simulink model "HPWnew"  (R2015a)
settings: Solver=ode45  StartTime=0.0  StopTime=10.0  RelTol=1e-3
undefined symbols (not defined in the file): c1, c2, c3, c4, c5, c6, Hydride, Metal, Nickel, PV1, PV2, PV3
libraries: powerlib x263, electricdrivelib x30, powerlib_meascontrol x15, powerlib_extras x7, re_lib x3, fuzblock x3, simulink x2
(part 1 of 8)
settings Model: Creator=Indhu  LastModifiedBy=Indhu
settings DebuggingCC: SolverPrmCheckMsg=warning

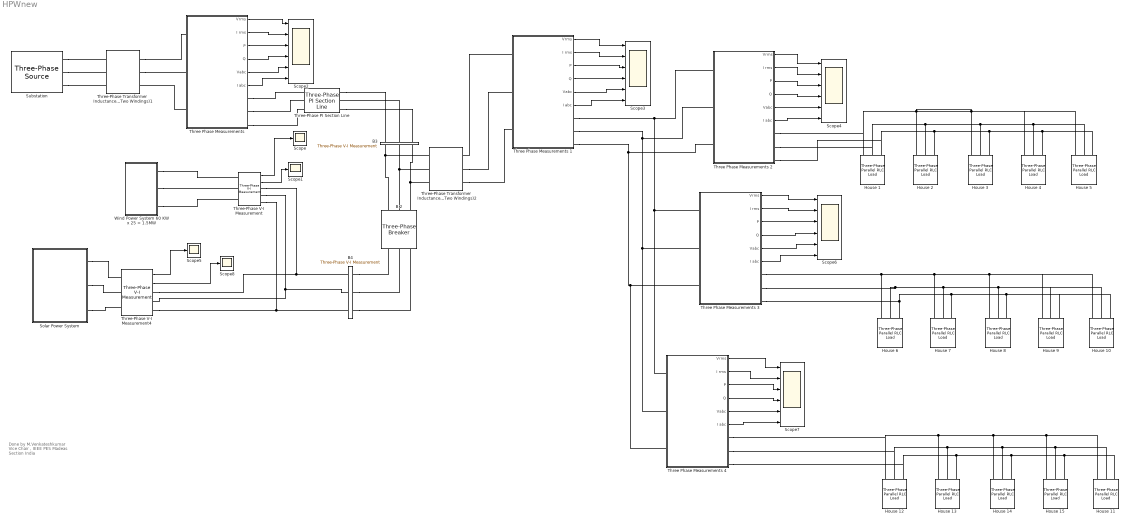
== system HPWnew ==
  note: Done by
      | M.Venkateshkumar
      | Vice Chair , IEEE PES
      | Madeas Section India
  B 2 : powerlib/Elements/Three-Phase Breaker  InitialState=closed  SwitchA=off  SwitchB=off  SwitchC=off  SwitchTimes=[0.001 0.3]  External=off  BreakerResistance=0.001  SnubberResistance=1e6  SnubberCapacitance=inf  Measurements=None
  B3 : powerlib/Measurements/Three-Phase V-I Measurement  VoltageMeasurement=phase-to-ground  SetLabelV=on  LabelV=Vabc_B3  Vpu=off  VpuLL=off  CurrentMeasurement=yes  SetLabelI=on  LabelI=A3  Ipu=off  Pbase=100e6  Vbase=440  OutputType=Magnitude  PhasorSimulation=off  PSBequivalent=0
  B4 : powerlib/Measurements/Three-Phase V-I Measurement  VoltageMeasurement=phase-to-phase  SetLabelV=on  LabelV=Vabc_B4  Vpu=off  VpuLL=off  CurrentMeasurement=yes  SetLabelI=on  LabelI=Iabc_B4  Ipu=off  Pbase=100e6  Vbase=440  OutputType=Magnitude  PhasorSimulation=off  PSBequivalent=0
  House {1..5} (5 alike) : powerlib/Elements/Three-Phase Parallel RLC Load  LConnTagsString=A|B|C  Configuration=Y (grounded)  NominalVoltage=440  NominalFrequency=50  ActivePower=10e2  InductivePower=100  CapacitivePower=0  Measurements=None  LoadType=constant Z
  House {6..10} (5 alike) : powerlib/Elements/Three-Phase Parallel RLC Load  LConnTagsString=A|B|C  Configuration=Y (grounded)  NominalVoltage=440  NominalFrequency=50  ActivePower=10e3  InductivePower=100  CapacitivePower=0  Measurements=None  LoadType=constant Z
  House {11..15} (5 alike) : powerlib/Elements/Three-Phase Parallel RLC Load  LConnTagsString=A|B|C  Configuration=Y (grounded)  NominalVoltage=440  NominalFrequency=50  ActivePower=50e3  InductivePower=100  CapacitivePower=0  Measurements=None  LoadType=constant Z
  Scope{,1,5,8} (4 alike) : Scope
      Scope settings: YMin=-750  YMax=750
      Scope1 settings: YMin=-250  YMax=250  SaveName=ScopeData2
      Scope5 settings: YMin=-600  YMax=550  SaveName=ScopeData8
      Scope8 settings: SaveName=ScopeData9
  Scope{2..4,6..7} (5 alike) : Scope  NumInputPorts=6
      Scope2 settings: TimeRange=1.6  YMin=100~50~-100000~-100000~-500~-500  YMax=300~200~100000~100000~500~500  SaveName=ScopeData3
      Scope3 settings: TimeRange=1.6  YMin=100~50~-100000~-100000~-500~-500  YMax=300~200~100000~100000~500~500  SaveName=ScopeData4
      Scope4 settings: TimeRange=1.6  YMin=100~50~-100000~-100000~-500~-500  YMax=300~200~100000~100000~500~500  SaveName=ScopeData6
      Scope6 settings: TimeRange=1.6  YMin=100~50~-100000~-100000~-500~-500  YMax=300~200~100000~100000~500~500  SaveName=ScopeData7
      Scope7 settings: TimeRange=1.6  YMin=100~50~-100000~-100000~-500~-500  YMax=300~200~100000~100000~500~500  SaveName=ScopeData10
  "Solar Power System " : Subsystem
  "Substation " : powerlib/Electrical Sources/Three-Phase Source  Voltage=(25000)*1.00008  PhaseAngle=0.13223  Frequency=50  InternalConnection=Yg  SpecifyImpedance=on  Resistance=0.8929  Inductance=16.58e-3  ShortCircuitLevel=100e6  BaseVoltage=63510.4  XRratio=7  BusType=swing  Pref=0  Qref=0  Qmin=-inf  Qmax=inf
  "Three Phase Measurements " : Subsystem
  Three Phase Measurements 1 : Subsystem
  Three Phase Measurements 2 : Subsystem
  Three Phase Measurements 3 : Subsystem
  Three Phase Measurements 4 : Subsystem
  Three-Phase PI Section Line : powerlib/Elements/Three-Phase PI Section Line  LConnTagsString=a|b|c  RConnTagsString=A|B|C  Frequency=50  Resistances=[ 0.01273 0.3864]  Inductances="[ 0.9337e-3  4.1264e-3]"  Capacitances=[12.74e-9 7.751e-9]  Length=10
  Three-Phase V-I Measurement : powerlib/Measurements/Three-Phase V-I Measurement  VoltageMeasurement=phase-to-ground  SetLabelV=off  LabelV=Vabc  Vpu=off  VpuLL=off  CurrentMeasurement=yes  SetLabelI=off  LabelI=Iabc  Ipu=off  Pbase=100e6  Vbase=500e3  OutputType=Complex  PhasorSimulation=off  PSBequivalent=0
  Three-Phase V-I Measurement4 : powerlib/Measurements/Three-Phase V-I Measurement  VoltageMeasurement=phase-to-ground  SetLabelV=off  LabelV=Vabc  Vpu=off  VpuLL=off  CurrentMeasurement=yes  SetLabelI=off  LabelI=Iabc  Ipu=off  Pbase=100e6  Vbase=500e3  OutputType=Complex  PhasorSimulation=off  PSBequivalent=0
  Three-Phase Transformer Inductance Matrix Type (Two Windings)1 : powerlib/Elements/Three-Phase Transformer Inductance Matrix Type (Two Windings)  CoreType=Three-limb or five-limb core  Winding1Connection=Yg  Winding2Connection=Yg  AutoTransformer=off  Measurements=None  NominalPower=[100e3 50]  VLLnom=[63510.4 600]  WindingResistances=[0.01 0.01]  NoLoadIexcPos=2  NoLoadPlossPos=1000  ShortCircuitReactancePos=0.06  ShortCircuitReactancePosAuto=0.06  NoLoadIexcZero=100  NoLoadPlossZero=1500  ShortCircuitReactanceZero=0.03  ShortCircuitReactanceZeroAuto=0.03
  Three-Phase Transformer Inductance Matrix Type (Two Windings)2 : powerlib/Elements/Three-Phase Transformer Inductance Matrix Type (Two Windings)  CoreType=Three-limb or five-limb core  Winding1Connection=Yg  Winding2Connection=Yg  AutoTransformer=off  Measurements=None  NominalPower=[100e3 50]  VLLnom=[63510.4 600]  WindingResistances=[0.01 0.01]  NoLoadIexcPos=2  NoLoadPlossPos=1000  ShortCircuitReactancePos=0.06  ShortCircuitReactancePosAuto=0.06  NoLoadIexcZero=100  NoLoadPlossZero=1500  ShortCircuitReactanceZero=0.03  ShortCircuitReactanceZeroAuto=0.03
  Wind Power System 60 KW x 25 = 1.5MW : Subsystem
  wires:
  Three-Phase V-I Measurement/1 -> Scope/1
  Three-Phase V-I Measurement/2 -> Scope1/1
  Three-Phase V-I Measurement4/1 -> Scope5/1
  Three-Phase V-I Measurement4/2 -> Scope8/1
  "Three Phase Measurements "/3(P) -> Scope2/3
  "Three Phase Measurements "/4(Q) -> Scope2/4
  "Three Phase Measurements "/2(I rms) -> Scope2/2
  "Three Phase Measurements "/5(Vabc) -> Scope2/5
  "Three Phase Measurements "/1(Vrms) -> Scope2/1
  "Three Phase Measurements "/6(I abc) -> Scope2/6
  Three Phase Measurements 1/3(P) -> Scope3/3
  Three Phase Measurements 1/4(Q) -> Scope3/4
  Three Phase Measurements 1/2(I rms) -> Scope3/2
  Three Phase Measurements 1/5(Vabc) -> Scope3/5
  Three Phase Measurements 1/1(Vrms) -> Scope3/1
  Three Phase Measurements 1/6(I abc) -> Scope3/6
  Three Phase Measurements 2/3(P) -> Scope4/3
  Three Phase Measurements 2/4(Q) -> Scope4/4
  Three Phase Measurements 2/2(I rms) -> Scope4/2
  Three Phase Measurements 2/5(Vabc) -> Scope4/5
  Three Phase Measurements 2/1(Vrms) -> Scope4/1
  Three Phase Measurements 2/6(I abc) -> Scope4/6
  Three Phase Measurements 3/3(P) -> Scope6/3
  Three Phase Measurements 3/4(Q) -> Scope6/4
  Three Phase Measurements 3/2(I rms) -> Scope6/2
  Three Phase Measurements 3/5(Vabc) -> Scope6/5
  Three Phase Measurements 3/1(Vrms) -> Scope6/1
  Three Phase Measurements 3/6(I abc) -> Scope6/6
  Three Phase Measurements 4/3(P) -> Scope7/3
  Three Phase Measurements 4/4(Q) -> Scope7/4
  Three Phase Measurements 4/2(I rms) -> Scope7/2
  Three Phase Measurements 4/5(Vabc) -> Scope7/5
  Three Phase Measurements 4/1(Vrms) -> Scope7/1
  Three Phase Measurements 4/6(I abc) -> Scope7/6
  connections:
  B 2/LConn1 -- Three-Phase Transformer Inductance Matrix Type (Two Windings)2/LConn1 -- B3/LConn1
  B 2/LConn2 -- Three-Phase Transformer Inductance Matrix Type (Two Windings)2/LConn2 -- B3/LConn2
  B 2/LConn3 -- Three-Phase Transformer Inductance Matrix Type (Two Windings)2/LConn3 -- B3/LConn3
  B4/LConn3 -- B 2/RConn3
  B4/LConn1 -- B 2/RConn1
  B4/LConn2 -- B 2/RConn2
  "Solar Power System "/RConn2 -- Three-Phase V-I Measurement4/LConn2
  "Solar Power System "/RConn3 -- Three-Phase V-I Measurement4/LConn3
  "Solar Power System "/RConn1 -- Three-Phase V-I Measurement4/LConn1
  "Three Phase Measurements "/LConn3 -- Three-Phase Transformer Inductance Matrix Type (Two Windings)1/RConn3
  Three-Phase Transformer Inductance Matrix Type (Two Windings)1/RConn2 -- "Three Phase Measurements "/LConn2
  Three-Phase Transformer Inductance Matrix Type (Two Windings)1/RConn1 -- "Three Phase Measurements "/LConn1
  "Substation "/RConn1 -- Three-Phase Transformer Inductance Matrix Type (Two Windings)1/LConn1
  "Substation "/RConn2 -- Three-Phase Transformer Inductance Matrix Type (Two Windings)1/LConn2
  "Substation "/RConn3 -- Three-Phase Transformer Inductance Matrix Type (Two Windings)1/LConn3
  Three-Phase PI Section Line/RConn1 -- B3/RConn1
  B3/RConn2 -- Three-Phase PI Section Line/RConn2
  Three-Phase PI Section Line/RConn3 -- B3/RConn3
  Three-Phase V-I Measurement/RConn1 -- Three-Phase V-I Measurement4/RConn1 -- B4/RConn1
  Three-Phase V-I Measurement/RConn2 -- Three-Phase V-I Measurement4/RConn2 -- B4/RConn2
  Three-Phase V-I Measurement/RConn3 -- Three-Phase V-I Measurement4/RConn3 -- B4/RConn3
  House 4/LConn1 -- House 5/LConn1 -- House 3/LConn1 -- House 1/LConn1 -- Three Phase Measurements 2/RConn1 -- House 2/LConn1
  House 11/LConn2 -- House 15/LConn2 -- House 14/LConn2 -- Three Phase Measurements 4/RConn2 -- House 12/LConn2 -- House 13/LConn2
  House 11/LConn3 -- House 15/LConn3 -- House 14/LConn3 -- Three Phase Measurements 4/RConn3 -- House 12/LConn3 -- House 13/LConn3
  "Three Phase Measurements "/RConn1 -- Three-Phase PI Section Line/LConn1
  "Three Phase Measurements "/RConn2 -- Three-Phase PI Section Line/LConn2
  "Three Phase Measurements "/RConn3 -- Three-Phase PI Section Line/LConn3
  Three-Phase Transformer Inductance Matrix Type (Two Windings)2/RConn1 -- Three Phase Measurements 1/LConn1
  Three-Phase Transformer Inductance Matrix Type (Two Windings)2/RConn2 -- Three Phase Measurements 1/LConn2
  Three-Phase Transformer Inductance Matrix Type (Two Windings)2/RConn3 -- Three Phase Measurements 1/LConn3
  Wind Power System 60 KW x 25 = 1.5MW/RConn2 -- Three-Phase V-I Measurement/LConn2
  Wind Power System 60 KW x 25 = 1.5MW/RConn1 -- Three-Phase V-I Measurement/LConn1
  Wind Power System 60 KW x 25 = 1.5MW/RConn3 -- Three-Phase V-I Measurement/LConn3
  House 4/LConn3 -- House 1/LConn3 -- Three Phase Measurements 2/RConn3 -- House 2/LConn3 -- House 3/LConn3 -- House 5/LConn3
  House 4/LConn2 -- House 1/LConn2 -- Three Phase Measurements 2/RConn2 -- House 2/LConn2 -- House 3/LConn2 -- House 5/LConn2
  House 8/LConn1 -- House 10/LConn1 -- House 9/LConn1 -- House 7/LConn1 -- House 6/LConn1 -- Three Phase Measurements 3/RConn1
  House 7/LConn2 -- House 8/LConn2 -- House 10/LConn2 -- House 9/LConn2 -- Three Phase Measurements 3/RConn2 -- House 6/LConn2
  House 15/LConn1 -- House 11/LConn1 -- House 14/LConn1 -- Three Phase Measurements 4/RConn1 -- House 12/LConn1 -- House 13/LConn1
  House 7/LConn3 -- House 8/LConn3 -- House 10/LConn3 -- House 9/LConn3 -- House 6/LConn3 -- Three Phase Measurements 3/RConn3
  Three Phase Measurements 3/LConn1 -- Three Phase Measurements 2/LConn1 -- Three Phase Measurements 1/RConn1 -- Three Phase Measurements 4/LConn1
  Three Phase Measurements 3/LConn2 -- Three Phase Measurements 2/LConn2 -- Three Phase Measurements 1/RConn2 -- Three Phase Measurements 4/LConn2
  Three Phase Measurements 3/LConn3 -- Three Phase Measurements 4/LConn3 -- Three Phase Measurements 2/LConn3 -- Three Phase Measurements 1/RConn3

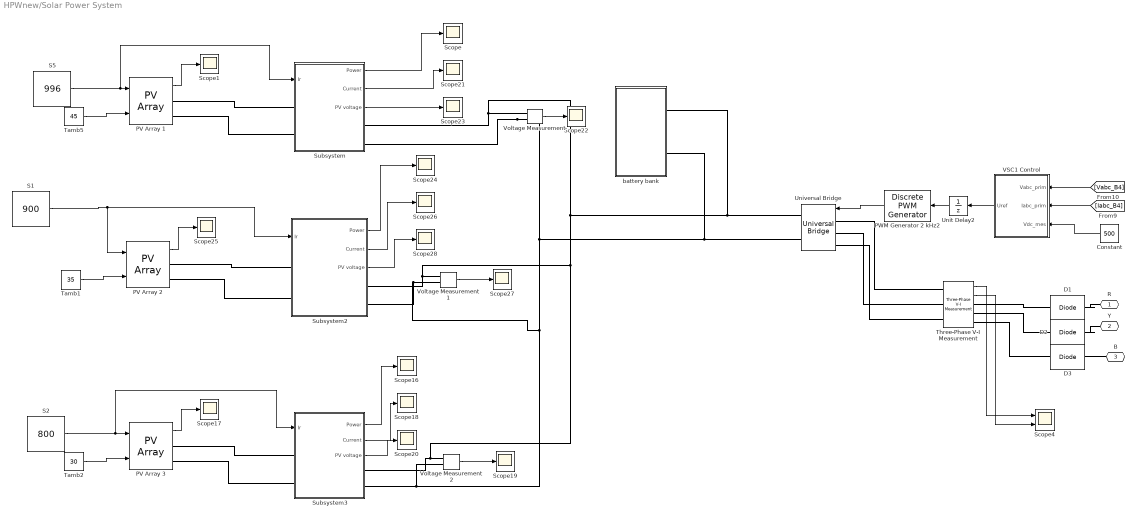
== system HPWnew/Solar Power System  ==
  Constant : Constant  Value=500
  D1 : powerlib/Power Electronics/Diode  Ron=0.001  Lon=0  Vf=0.1  IC=0  UseSnubber=off  Rs=50000  Cs=250e-12  Measurements=off
  D2 : powerlib/Power Electronics/Diode  Ron=0.001  Lon=0  Vf=0.1  IC=0  UseSnubber=off  Rs=50000  Cs=250e-12  Measurements=off
  D3 : powerlib/Power Electronics/Diode  Ron=0.001  Lon=0  Vf=0.1  IC=0  UseSnubber=off  Rs=50000  Cs=250e-12  Measurements=off
  PV Array 1 : re_lib/Solar/PV Array  Npar=3  Nser=1  PlotType=array @ 25 deg.C & specified irradiances  S_vec="[ 1000  500  100 ]"  Temp_C_vec="[ 45 25  ]"  ModuleName=User-defined  PlotWhenSelected=on  Pm=276.21  Ncell=36  Voc=41.8  Isc=7.4  Vm=40.5  Im=6.82  beta_Voc_pc=-0.365  alpha_Isc_pc=0.0445  beta_Voc=-0.15257  alpha_Isc=0.003293  IL=7.4001  I0=1.6325e-15  nI=1.3667  Rsh=139.6555  Rs=0.080363  BAL=off  Tc=1e-6  Tfilter=10
  PV Array 2 : re_lib/Solar/PV Array  Npar=3  Nser=1  PlotType=array @ 25 deg.C & specified irradiances  S_vec="[ 1000  500  100 ]"  Temp_C_vec="[ 45 25  ]"  ModuleName=User-defined  PlotWhenSelected=on  Pm=276.21  Ncell=36  Voc=41.8  Isc=7.4  Vm=40.5  Im=6.82  beta_Voc_pc=-0.365  alpha_Isc_pc=0.0445  beta_Voc=-0.15257  alpha_Isc=0.003293  IL=7.4001  I0=1.6325e-15  nI=1.3667  Rsh=139.6555  Rs=0.080363  BAL=off  Tc=1e-6  Tfilter=10
  PV Array 3 : re_lib/Solar/PV Array  Npar=3  Nser=1  PlotType=array @ 25 deg.C & specified irradiances  S_vec="[ 1000  500  100 ]"  Temp_C_vec="[ 45 25  ]"  ModuleName=User-defined  PlotWhenSelected=on  Pm=276.21  Ncell=36  Voc=41.8  Isc=7.4  Vm=40.5  Im=6.82  beta_Voc_pc=-0.365  alpha_Isc_pc=0.0445  beta_Voc=-0.15257  alpha_Isc=0.003293  IL=7.4001  I0=1.6325e-15  nI=1.3667  Rsh=139.6555  Rs=0.080363  BAL=off  Tc=1e-6  Tfilter=10
  PWM Generator 2 kHz2 : powerlib_extras/Discrete  Control Blocks/Discrete PWM Generator  GeneratorMode="3-arm  bridge (6 pulses)"  Fc=33*50  Ts=1  Internal=off  mIndex=0.4  Freq=60  Phase=0
  S1 : Constant  Value=900
  S2 : Constant  Value=800
  S5 : Constant  Value=996
  Scope{,1,16..28} (15 alike) : Scope
      Scope settings: YMin=1000  YMax=2200  SaveName=ScopeData5
      Scope1 settings: YMin=3.1175  YMax=3.145  SaveName=ScopeData24  MaxDataPoints=50000000
      Scope16 settings: YMin=-125  YMax=175  SaveName=ScopeData19
      Scope17 settings: YMin=3.1175  YMax=3.145  SaveName=ScopeData20  MaxDataPoints=50000000
      Scope18 settings: YMin=1.845  YMax=1.857  SaveName=ScopeData21
      Scope19 settings: YMin=190.2  YMax=191.4  SaveName=ScopeData22
      Scope20 settings: YMin=34.5  YMax=41  SaveName=ScopeData23
      Scope21 settings: YMin=1.845  YMax=1.857  SaveName=ScopeData25
      Scope22 settings: YMin=499.8  YMax=500.2  SaveName=ScopeData26
      Scope23 settings: YMin=0  YMax=225  SaveName=ScopeData27
      Scope24 settings: YMin=-1000  YMax=10000  SaveName=ScopeData28
      Scope25 settings: YMin=3.1175  YMax=3.145  SaveName=ScopeData29  MaxDataPoints=50000000
      Scope26 settings: YMin=1.845  YMax=1.857  SaveName=ScopeData30
      Scope27 settings: YMin=499.8  YMax=500.2  SaveName=ScopeData31
      Scope28 settings: YMin=0  YMax=200  SaveName=ScopeData18
  Scope4 : Scope  NumInputPorts=2
      settings: ShowLegends=on  YMin=-950~-0.025  YMax=-100~0.5  SaveName=MLFCDSTAT
  Subsystem : Subsystem
  Subsystem2 : Subsystem
  Subsystem3 : Subsystem
  Tamb1 : Constant  Value=35
  Tamb2 : Constant  Value=30
  Tamb5 : Constant  Value=45
  Three-Phase V-I Measurement : powerlib/Measurements/Three-Phase V-I Measurement  VoltageMeasurement=phase-to-ground  SetLabelV=off  LabelV=Vabc  Vpu=off  VpuLL=off  CurrentMeasurement=yes  SetLabelI=off  LabelI=Iabc  Ipu=off  Pbase=100e6  Vbase=500e3  OutputType=Complex  PhasorSimulation=off  PSBequivalent=0
  Unit Delay2 : UnitDelay
  Universal Bridge : powerlib/Power Electronics/Universal Bridge  Arms=3  SnubberResistance=1e5  SnubberCapacitance=inf  Device=MOSFET / Diodes  Ron=1e-3  Lon=0  ForwardVoltages="[  0  0  ]"  ForwardVoltage=0  GTOparameters=[ 10e-6 , 20e-6 ]  IGBTparameters=[ 1e-6 , 2e-6 ]  Measurements=None  Measurements_2=None  converterType=Rectifier
  VSC1 Control : Subsystem  mask(VSC Main Controller){nom=[ 50e3  50 ], Vnom=[ 6350.9 254.03 ], Vnom_dc=500, RLxfo=[0.008  0.04 ], RLchoke=[2e-3*(2*pi*60)/50   2e-3], K_VDCreg=[7  800], K_Ireg=[0.3 20]*1.5, Ts=1}
      mask prompts: nom "Nominal power and frequency [ Pnom(VA)  Fnom(Hz) ]:"; Vnom "Nominal primary and secondary voltages (Vrms LL) [ Vnom_prim   Vnom_sec ]:"; Vnom_dc "Nominal DC bus voltage (V):"; RLxfo "Total transformer leakage impedance (pu/Pnom) [ Rxfo  Lxf ]"; RLchoke "Choke impedance [ R(ohm) L(H) ]"; K_VDCreg "VDC regultator gains [ Kp  Ki ]:"; K_Ireg "Current regulator gains [ Kp  Ki ]:"; Ts "Sample time"
      mask init:
      | Pnom=nom(1);
      | Fnom=nom(2);
      | Vnom_prim=Vnom(1);
      | Vnom_sec=Vnom(2);
      | Zbase=Vnom_sec^2/Pnom;
      | Rtot_pu=RLxfo(1) + RLchoke(1)/Zbase;
      | Ltot_pu=RLxfo(2) + RLchoke(2)/(Zbase/(2*pi*Fnom));
      | Kp_VDCreg=K_VDCreg(1);
      | Ki_VDCreg=K_VDCreg(2);
      | Kp_Ireg=K_Ireg(1);
      | Ki_Ireg=K_Ireg(2);
      | Vdc_ref=Vnom_dc;
      | % Used to determine initial value of Boost Control (MPPT)
      | assignin('base','Vdc_ref_Inv',Vdc_ref);
  Voltage Measurement : powerlib/Measurements/Voltage Measurement  PhasorSimulation=off  OutputType=Complex  PSBequivalent=0
  Voltage Measurement1 : powerlib/Measurements/Voltage Measurement  PhasorSimulation=off  OutputType=Complex  PSBequivalent=0
  Voltage Measurement2 : powerlib/Measurements/Voltage Measurement  PhasorSimulation=off  OutputType=Complex  PSBequivalent=0
  "battery bank " : Subsystem
  R : PMIOPort  Port=1  Side=Right
  Y : PMIOPort  Port=2  Side=Right
  B : PMIOPort  Port=3  Side=Right
  wires:
  [Vabc_B4] -> VSC1 Control/1(Vabc_prim)
  [Iabc_B4] -> VSC1 Control/2(Iabc_prim)
  PWM Generator 2 kHz2/1 -> Universal Bridge/1
  Constant/1 -> VSC1 Control/3(Vdc_mes)
  Three-Phase V-I Measurement/1 -> Scope4/1
  Three-Phase V-I Measurement/2 -> Scope4/2
  Unit Delay2/1 -> PWM Generator 2 kHz2/1
  VSC1 Control/1(Uref) -> Unit Delay2/1
  Tamb5/1 -> PV Array 1/2
  PV Array 1/1 -> Scope1/1
  Subsystem/1(Power) -> Scope/1
  Subsystem/2("Current ") -> Scope21/1
  Voltage Measurement/1 -> Scope22/1
  Subsystem/3("PV voltage ") -> Scope23/1
  S1/1 -> Subsystem2/1(Ir), PV Array 2/1
  Tamb1/1 -> PV Array 2/2
  PV Array 2/1 -> Scope25/1
  Subsystem2/1(Power) -> Scope24/1
  Subsystem2/2("Current ") -> Scope26/1
  Voltage Measurement1/1 -> Scope27/1
  Subsystem2/3("PV voltage ") -> Scope28/1
  Tamb2/1 -> PV Array 3/2
  PV Array 3/1 -> Scope17/1
  Subsystem3/1(Power) -> Scope16/1
  Subsystem3/2("Current ") -> Scope18/1
  Voltage Measurement2/1 -> Scope19/1
  Subsystem3/3("PV voltage ") -> Scope20/1
  S5/1 -> Subsystem/1(Ir), PV Array 1/1
  S2/1 -> Subsystem3/1(Ir), PV Array 3/1
  connections:
  Three-Phase V-I Measurement/LConn1 -- Universal Bridge/LConn1
  Three-Phase V-I Measurement/LConn2 -- Universal Bridge/LConn2
  Three-Phase V-I Measurement/RConn2 -- D2/LConn1
  D3/RConn1 -- B/RConn1
  D2/RConn1 -- Y/RConn1
  Three-Phase V-I Measurement/LConn3 -- Universal Bridge/LConn3
  Three-Phase V-I Measurement/RConn1 -- D1/LConn1
  D1/RConn1 -- R/RConn1
  Three-Phase V-I Measurement/RConn3 -- D3/LConn1
  Voltage Measurement2/LConn1 -- Subsystem3/RConn1 -- "battery bank "/RConn1 -- Universal Bridge/RConn1 -- Subsystem/RConn1 -- Voltage Measurement/LConn1 -- Subsystem2/RConn1 -- Voltage Measurement1/LConn1
  Subsystem3/RConn2 -- Voltage Measurement2/LConn2 -- "battery bank "/RConn2 -- Universal Bridge/RConn2 -- Subsystem/RConn2 -- Voltage Measurement/LConn2 -- Subsystem2/RConn2 -- Voltage Measurement1/LConn2
  PV Array 2/RConn2 -- Subsystem2/LConn2
  PV Array 2/RConn1 -- Subsystem2/LConn1
  PV Array 1/RConn2 -- Subsystem/LConn2
  PV Array 1/RConn1 -- Subsystem/LConn1
  PV Array 3/RConn2 -- Subsystem3/LConn2
  PV Array 3/RConn1 -- Subsystem3/LConn1

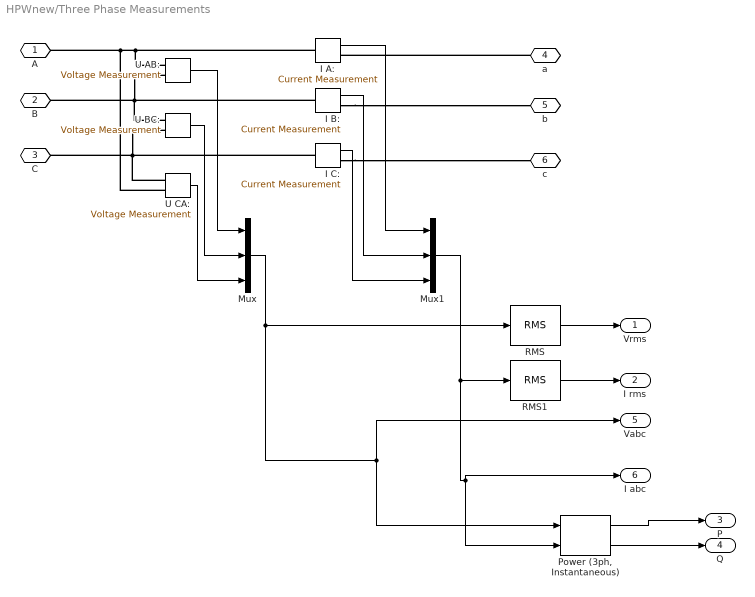
== system HPWnew/Three Phase Measurements  ==
  I A: : powerlib/Measurements/Current Measurement  PhasorSimulation=off  OutputType=Complex  PSBequivalent=0
  I B: : powerlib/Measurements/Current Measurement  PhasorSimulation=off  OutputType=Complex  PSBequivalent=0
  I C: : powerlib/Measurements/Current Measurement  PhasorSimulation=off  OutputType=Complex  PSBequivalent=0
  Mux : Mux  Inputs=3
  Mux1 : Mux  Inputs=3
  "Power (3ph, Instantaneous)" : powerlib_meascontrol/Measurements/Power (3ph, Instantaneous)
  RMS : powerlib_meascontrol/Measurements/RMS  TrueRMS=on  Freq=60  RMSInit=120  Ts=0
  RMS1 : powerlib_meascontrol/Measurements/RMS  TrueRMS=on  Freq=60  RMSInit=120  Ts=0
  U AB: : powerlib/Measurements/Voltage Measurement  PhasorSimulation=off  OutputType=Complex  PSBequivalent=0
  U BC: : powerlib/Measurements/Voltage Measurement  PhasorSimulation=off  OutputType=Complex  PSBequivalent=0
  U CA: : powerlib/Measurements/Voltage Measurement  PhasorSimulation=off  OutputType=Complex  PSBequivalent=0
  A : PMIOPort  Port=1  Side=Left
  B : PMIOPort  Port=2  Side=Left
  C : PMIOPort  Port=3  Side=Left
  a : PMIOPort  Port=4  Side=Right
  b : PMIOPort  Port=5  Side=Right
  c : PMIOPort  Port=6  Side=Right
  Vrms : Outport
  I rms : Outport  Port=2
  P : Outport  Port=3
  Q : Outport  Port=4
  Vabc : Outport  Port=5
  I abc : Outport  Port=6
  wires:
  I A:/1 -> Mux1/1
  Mux/1 -> Vabc/1, "Power (3ph, Instantaneous)"/1, RMS/1
  I C:/1 -> Mux1/3
  I B:/1 -> Mux1/2
  "Power (3ph, Instantaneous)"/2 -> Q/1
  Mux1/1 -> "Power (3ph, Instantaneous)"/2, I abc/1, RMS1/1
  U CA:/1 -> Mux/3
  U AB:/1 -> Mux/1
  U BC:/1 -> Mux/2
  RMS1/1 -> I rms/1
  RMS/1 -> Vrms/1
  "Power (3ph, Instantaneous)"/1 -> P/1
  connections:
  I C:/RConn1 -- c/RConn1
  a/RConn1 -- I A:/RConn1
  U CA:/LConn2 -- I A:/LConn1 -- U AB:/LConn1 -- A/RConn1
  I C:/LConn1 -- U BC:/LConn2 -- U CA:/LConn1 -- C/RConn1
  I B:/LConn1 -- U AB:/LConn2 -- U BC:/LConn1 -- B/RConn1
  I B:/RConn1 -- b/RConn1

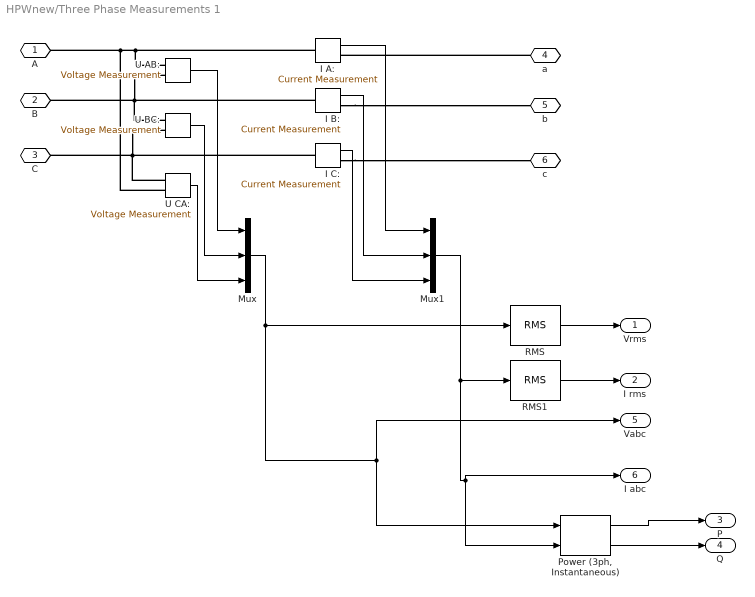
== system HPWnew/Three Phase Measurements 1 ==
  I A: : powerlib/Measurements/Current Measurement  PhasorSimulation=off  OutputType=Complex  PSBequivalent=0
  I B: : powerlib/Measurements/Current Measurement  PhasorSimulation=off  OutputType=Complex  PSBequivalent=0
  I C: : powerlib/Measurements/Current Measurement  PhasorSimulation=off  OutputType=Complex  PSBequivalent=0
  Mux : Mux  Inputs=3
  Mux1 : Mux  Inputs=3
  "Power (3ph, Instantaneous)" : powerlib_meascontrol/Measurements/Power (3ph, Instantaneous)
  RMS : powerlib_meascontrol/Measurements/RMS  TrueRMS=on  Freq=60  RMSInit=120  Ts=0
  RMS1 : powerlib_meascontrol/Measurements/RMS  TrueRMS=on  Freq=60  RMSInit=120  Ts=0
  U AB: : powerlib/Measurements/Voltage Measurement  PhasorSimulation=off  OutputType=Complex  PSBequivalent=0
  U BC: : powerlib/Measurements/Voltage Measurement  PhasorSimulation=off  OutputType=Complex  PSBequivalent=0
  U CA: : powerlib/Measurements/Voltage Measurement  PhasorSimulation=off  OutputType=Complex  PSBequivalent=0
  A : PMIOPort  Port=1  Side=Left
  B : PMIOPort  Port=2  Side=Left
  C : PMIOPort  Port=3  Side=Left
  a : PMIOPort  Port=4  Side=Right
  b : PMIOPort  Port=5  Side=Right
  c : PMIOPort  Port=6  Side=Right
  Vrms : Outport
  I rms : Outport  Port=2
  P : Outport  Port=3
  Q : Outport  Port=4
  Vabc : Outport  Port=5
  I abc : Outport  Port=6
  wires:
  "Power (3ph, Instantaneous)"/1 -> P/1
  RMS/1 -> Vrms/1
  RMS1/1 -> I rms/1
  U BC:/1 -> Mux/2
  U AB:/1 -> Mux/1
  U CA:/1 -> Mux/3
  Mux1/1 -> RMS1/1, I abc/1, "Power (3ph, Instantaneous)"/2
  "Power (3ph, Instantaneous)"/2 -> Q/1
  I B:/1 -> Mux1/2
  I C:/1 -> Mux1/3
  Mux/1 -> RMS/1, "Power (3ph, Instantaneous)"/1, Vabc/1
  I A:/1 -> Mux1/1
  connections:
  I B:/RConn1 -- b/RConn1
  B/RConn1 -- U BC:/LConn1 -- U AB:/LConn2 -- I B:/LConn1
  C/RConn1 -- U CA:/LConn1 -- U BC:/LConn2 -- I C:/LConn1
  A/RConn1 -- U AB:/LConn1 -- I A:/LConn1 -- U CA:/LConn2
  a/RConn1 -- I A:/RConn1
  I C:/RConn1 -- c/RConn1

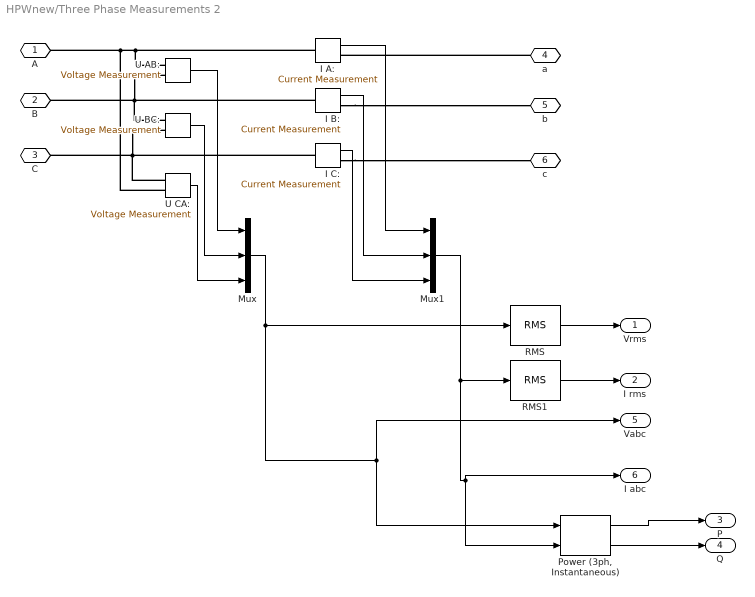
== system HPWnew/Three Phase Measurements 2 ==
  I A: : powerlib/Measurements/Current Measurement  PhasorSimulation=off  OutputType=Complex  PSBequivalent=0
  I B: : powerlib/Measurements/Current Measurement  PhasorSimulation=off  OutputType=Complex  PSBequivalent=0
  I C: : powerlib/Measurements/Current Measurement  PhasorSimulation=off  OutputType=Complex  PSBequivalent=0
  Mux : Mux  Inputs=3
  Mux1 : Mux  Inputs=3
  "Power (3ph, Instantaneous)" : powerlib_meascontrol/Measurements/Power (3ph, Instantaneous)
  RMS : powerlib_meascontrol/Measurements/RMS  TrueRMS=on  Freq=60  RMSInit=120  Ts=0
  RMS1 : powerlib_meascontrol/Measurements/RMS  TrueRMS=on  Freq=60  RMSInit=120  Ts=0
  U AB: : powerlib/Measurements/Voltage Measurement  PhasorSimulation=off  OutputType=Complex  PSBequivalent=0
  U BC: : powerlib/Measurements/Voltage Measurement  PhasorSimulation=off  OutputType=Complex  PSBequivalent=0
  U CA: : powerlib/Measurements/Voltage Measurement  PhasorSimulation=off  OutputType=Complex  PSBequivalent=0
  A : PMIOPort  Port=1  Side=Left
  B : PMIOPort  Port=2  Side=Left
  C : PMIOPort  Port=3  Side=Left
  a : PMIOPort  Port=4  Side=Right
  b : PMIOPort  Port=5  Side=Right
  c : PMIOPort  Port=6  Side=Right
  Vrms : Outport
  I rms : Outport  Port=2
  P : Outport  Port=3
  Q : Outport  Port=4
  Vabc : Outport  Port=5
  I abc : Outport  Port=6
  wires:
  I A:/1 -> Mux1/1
  Mux/1 -> Vabc/1, "Power (3ph, Instantaneous)"/1, RMS/1
  I C:/1 -> Mux1/3
  I B:/1 -> Mux1/2
  "Power (3ph, Instantaneous)"/2 -> Q/1
  Mux1/1 -> "Power (3ph, Instantaneous)"/2, I abc/1, RMS1/1
  U CA:/1 -> Mux/3
  U AB:/1 -> Mux/1
  U BC:/1 -> Mux/2
  RMS1/1 -> I rms/1
  RMS/1 -> Vrms/1
  "Power (3ph, Instantaneous)"/1 -> P/1
  connections:
  I C:/RConn1 -- c/RConn1
  a/RConn1 -- I A:/RConn1
  U CA:/LConn2 -- I A:/LConn1 -- U AB:/LConn1 -- A/RConn1
  I C:/LConn1 -- U BC:/LConn2 -- U CA:/LConn1 -- C/RConn1
  I B:/LConn1 -- U AB:/LConn2 -- U BC:/LConn1 -- B/RConn1
  I B:/RConn1 -- b/RConn1

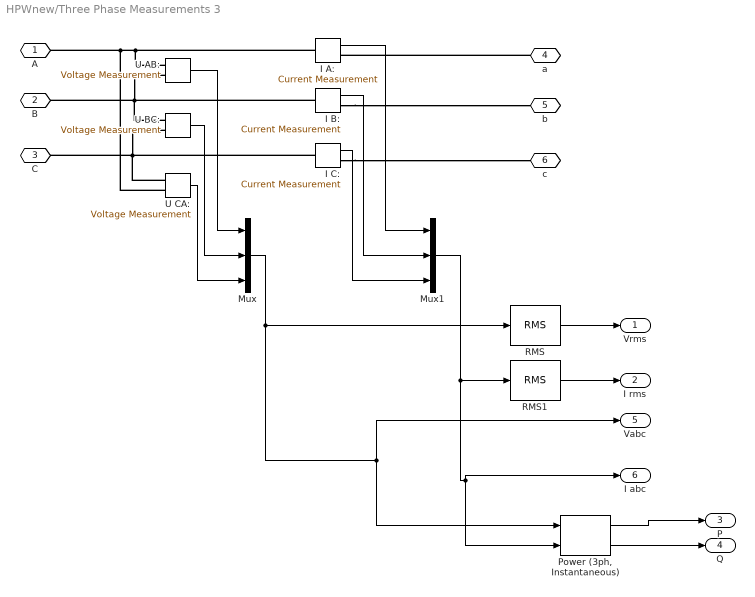
== system HPWnew/Three Phase Measurements 3 ==
  I A: : powerlib/Measurements/Current Measurement  PhasorSimulation=off  OutputType=Complex  PSBequivalent=0
  I B: : powerlib/Measurements/Current Measurement  PhasorSimulation=off  OutputType=Complex  PSBequivalent=0
  I C: : powerlib/Measurements/Current Measurement  PhasorSimulation=off  OutputType=Complex  PSBequivalent=0
  Mux : Mux  Inputs=3
  Mux1 : Mux  Inputs=3
  "Power (3ph, Instantaneous)" : powerlib_meascontrol/Measurements/Power (3ph, Instantaneous)
  RMS : powerlib_meascontrol/Measurements/RMS  TrueRMS=on  Freq=60  RMSInit=120  Ts=0
  RMS1 : powerlib_meascontrol/Measurements/RMS  TrueRMS=on  Freq=60  RMSInit=120  Ts=0
  U AB: : powerlib/Measurements/Voltage Measurement  PhasorSimulation=off  OutputType=Complex  PSBequivalent=0
  U BC: : powerlib/Measurements/Voltage Measurement  PhasorSimulation=off  OutputType=Complex  PSBequivalent=0
  U CA: : powerlib/Measurements/Voltage Measurement  PhasorSimulation=off  OutputType=Complex  PSBequivalent=0
  A : PMIOPort  Port=1  Side=Left
  B : PMIOPort  Port=2  Side=Left
  C : PMIOPort  Port=3  Side=Left
  a : PMIOPort  Port=4  Side=Right
  b : PMIOPort  Port=5  Side=Right
  c : PMIOPort  Port=6  Side=Right
  Vrms : Outport
  I rms : Outport  Port=2
  P : Outport  Port=3
  Q : Outport  Port=4
  Vabc : Outport  Port=5
  I abc : Outport  Port=6
  wires:
  "Power (3ph, Instantaneous)"/1 -> P/1
  RMS/1 -> Vrms/1
  RMS1/1 -> I rms/1
  U BC:/1 -> Mux/2
  U AB:/1 -> Mux/1
  U CA:/1 -> Mux/3
  Mux1/1 -> RMS1/1, I abc/1, "Power (3ph, Instantaneous)"/2
  "Power (3ph, Instantaneous)"/2 -> Q/1
  I B:/1 -> Mux1/2
  I C:/1 -> Mux1/3
  Mux/1 -> RMS/1, "Power (3ph, Instantaneous)"/1, Vabc/1
  I A:/1 -> Mux1/1
  connections:
  I B:/RConn1 -- b/RConn1
  B/RConn1 -- U BC:/LConn1 -- U AB:/LConn2 -- I B:/LConn1
  C/RConn1 -- U CA:/LConn1 -- U BC:/LConn2 -- I C:/LConn1
  A/RConn1 -- U AB:/LConn1 -- I A:/LConn1 -- U CA:/LConn2
  a/RConn1 -- I A:/RConn1
  I C:/RConn1 -- c/RConn1

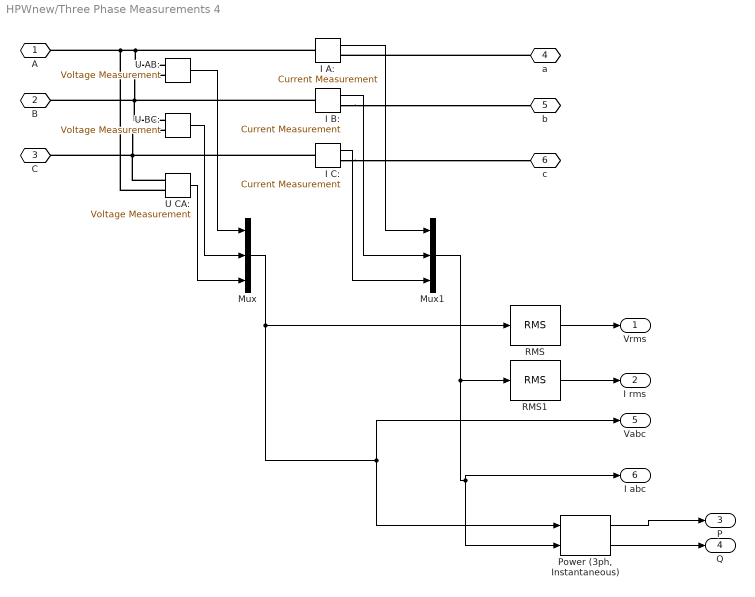
== system HPWnew/Three Phase Measurements 4 ==
  I A: : powerlib/Measurements/Current Measurement  PhasorSimulation=off  OutputType=Complex  PSBequivalent=0
  I B: : powerlib/Measurements/Current Measurement  PhasorSimulation=off  OutputType=Complex  PSBequivalent=0
  I C: : powerlib/Measurements/Current Measurement  PhasorSimulation=off  OutputType=Complex  PSBequivalent=0
  Mux : Mux  Inputs=3
  Mux1 : Mux  Inputs=3
  "Power (3ph, Instantaneous)" : powerlib_meascontrol/Measurements/Power (3ph, Instantaneous)
  RMS : powerlib_meascontrol/Measurements/RMS  TrueRMS=on  Freq=60  RMSInit=120  Ts=0
  RMS1 : powerlib_meascontrol/Measurements/RMS  TrueRMS=on  Freq=60  RMSInit=120  Ts=0
  U AB: : powerlib/Measurements/Voltage Measurement  PhasorSimulation=off  OutputType=Complex  PSBequivalent=0
  U BC: : powerlib/Measurements/Voltage Measurement  PhasorSimulation=off  OutputType=Complex  PSBequivalent=0
  U CA: : powerlib/Measurements/Voltage Measurement  PhasorSimulation=off  OutputType=Complex  PSBequivalent=0
  A : PMIOPort  Port=1  Side=Left
  B : PMIOPort  Port=2  Side=Left
  C : PMIOPort  Port=3  Side=Left
  a : PMIOPort  Port=4  Side=Right
  b : PMIOPort  Port=5  Side=Right
  c : PMIOPort  Port=6  Side=Right
  Vrms : Outport
  I rms : Outport  Port=2
  P : Outport  Port=3
  Q : Outport  Port=4
  Vabc : Outport  Port=5
  I abc : Outport  Port=6
  wires:
  I A:/1 -> Mux1/1
  Mux/1 -> Vabc/1, "Power (3ph, Instantaneous)"/1, RMS/1
  I C:/1 -> Mux1/3
  I B:/1 -> Mux1/2
  "Power (3ph, Instantaneous)"/2 -> Q/1
  Mux1/1 -> "Power (3ph, Instantaneous)"/2, I abc/1, RMS1/1
  U CA:/1 -> Mux/3
  U AB:/1 -> Mux/1
  U BC:/1 -> Mux/2
  RMS1/1 -> I rms/1
  RMS/1 -> Vrms/1
  "Power (3ph, Instantaneous)"/1 -> P/1
  connections:
  I C:/RConn1 -- c/RConn1
  a/RConn1 -- I A:/RConn1
  U CA:/LConn2 -- I A:/LConn1 -- U AB:/LConn1 -- A/RConn1
  I C:/LConn1 -- U BC:/LConn2 -- U CA:/LConn1 -- C/RConn1
  I B:/LConn1 -- U AB:/LConn2 -- U BC:/LConn1 -- B/RConn1
  I B:/RConn1 -- b/RConn1

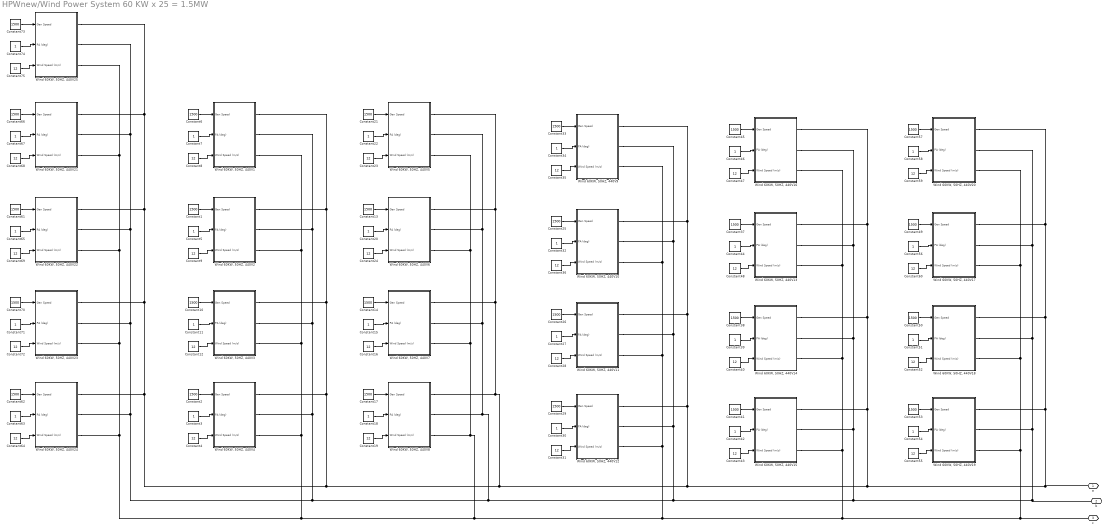
== system HPWnew/Wind Power System 60 KW x 25 = 1.5MW ==
  Constant{1..2,6,10,13..14,17,21,25..26,29,33,37..38,41,45,49..50,53,57,61..62,66,70,73} (25 alike) : Constant  Value=1500
  Constant{3,5,7,11,15,18,20,22,27,30,32,34,39,42,44,46,51,54,56,58,63,65,67,71,74} (25 alike) : Constant
  Constant{4,8..9,12,16,19,23..24,28,31,35..36,40,43,47..48,52,55,59..60,64,68..69,72,75} (25 alike) : Constant  Value=12
  "Wind 60KW, 50HZ, 440V1" : Subsystem
  "Wind 60KW, 50HZ, 440V10" : Subsystem
  "Wind 60KW, 50HZ, 440V11" : Subsystem
  "Wind 60KW, 50HZ, 440V12" : Subsystem
  "Wind 60KW, 50HZ, 440V13" : Subsystem
  "Wind 60KW, 50HZ, 440V14" : Subsystem
  "Wind 60KW, 50HZ, 440V15" : Subsystem
  "Wind 60KW, 50HZ, 440V16" : Subsystem
  "Wind 60KW, 50HZ, 440V17" : Subsystem
  "Wind 60KW, 50HZ, 440V18" : Subsystem
  "Wind 60KW, 50HZ, 440V19" : Subsystem
  "Wind 60KW, 50HZ, 440V2" : Subsystem
  "Wind 60KW, 50HZ, 440V20" : Subsystem
  "Wind 60KW, 50HZ, 440V21" : Subsystem
  "Wind 60KW, 50HZ, 440V22" : Subsystem
  "Wind 60KW, 50HZ, 440V23" : Subsystem
  "Wind 60KW, 50HZ, 440V24" : Subsystem
  "Wind 60KW, 50HZ, 440V25" : Subsystem
  "Wind 60KW, 50HZ, 440V3" : Subsystem
  "Wind 60KW, 50HZ, 440V4" : Subsystem
  "Wind 60KW, 50HZ, 440V5" : Subsystem
  "Wind 60KW, 50HZ, 440V6" : Subsystem
  "Wind 60KW, 50HZ, 440V7" : Subsystem
  "Wind 60KW, 50HZ, 440V8" : Subsystem
  "Wind 60KW, 50HZ, 440V9" : Subsystem
  a : PMIOPort  Port=1  Side=Right
  b : PMIOPort  Port=2  Side=Right
  c : PMIOPort  Port=3  Side=Right
  wires:
  Constant66/1 -> "Wind 60KW, 50HZ, 440V21"/1("Gen Speed ")
  Constant67/1 -> "Wind 60KW, 50HZ, 440V21"/2(PA (deg))
  Constant68/1 -> "Wind 60KW, 50HZ, 440V21"/3(Wind Speed (m/s))
  Constant61/1 -> "Wind 60KW, 50HZ, 440V22"/1("Gen Speed ")
  Constant65/1 -> "Wind 60KW, 50HZ, 440V22"/2(PA (deg))
  Constant69/1 -> "Wind 60KW, 50HZ, 440V22"/3(Wind Speed (m/s))
  Constant70/1 -> "Wind 60KW, 50HZ, 440V23"/1("Gen Speed ")
  Constant71/1 -> "Wind 60KW, 50HZ, 440V23"/2(PA (deg))
  Constant72/1 -> "Wind 60KW, 50HZ, 440V23"/3(Wind Speed (m/s))
  Constant62/1 -> "Wind 60KW, 50HZ, 440V24"/1("Gen Speed ")
  Constant63/1 -> "Wind 60KW, 50HZ, 440V24"/2(PA (deg))
  Constant64/1 -> "Wind 60KW, 50HZ, 440V24"/3(Wind Speed (m/s))
  Constant73/1 -> "Wind 60KW, 50HZ, 440V25"/1("Gen Speed ")
  Constant74/1 -> "Wind 60KW, 50HZ, 440V25"/2(PA (deg))
  Constant75/1 -> "Wind 60KW, 50HZ, 440V25"/3(Wind Speed (m/s))
  Constant6/1 -> "Wind 60KW, 50HZ, 440V1"/1("Gen Speed ")
  Constant7/1 -> "Wind 60KW, 50HZ, 440V1"/2(PA (deg))
  Constant8/1 -> "Wind 60KW, 50HZ, 440V1"/3(Wind Speed (m/s))
  Constant1/1 -> "Wind 60KW, 50HZ, 440V2"/1("Gen Speed ")
  Constant5/1 -> "Wind 60KW, 50HZ, 440V2"/2(PA (deg))
  Constant9/1 -> "Wind 60KW, 50HZ, 440V2"/3(Wind Speed (m/s))
  Constant10/1 -> "Wind 60KW, 50HZ, 440V3"/1("Gen Speed ")
  Constant11/1 -> "Wind 60KW, 50HZ, 440V3"/2(PA (deg))
  Constant12/1 -> "Wind 60KW, 50HZ, 440V3"/3(Wind Speed (m/s))
  Constant2/1 -> "Wind 60KW, 50HZ, 440V4"/1("Gen Speed ")
  Constant3/1 -> "Wind 60KW, 50HZ, 440V4"/2(PA (deg))
  Constant4/1 -> "Wind 60KW, 50HZ, 440V4"/3(Wind Speed (m/s))
  Constant21/1 -> "Wind 60KW, 50HZ, 440V5"/1("Gen Speed ")
  Constant22/1 -> "Wind 60KW, 50HZ, 440V5"/2(PA (deg))
  Constant23/1 -> "Wind 60KW, 50HZ, 440V5"/3(Wind Speed (m/s))
  Constant13/1 -> "Wind 60KW, 50HZ, 440V6"/1("Gen Speed ")
  Constant20/1 -> "Wind 60KW, 50HZ, 440V6"/2(PA (deg))
  Constant24/1 -> "Wind 60KW, 50HZ, 440V6"/3(Wind Speed (m/s))
  Constant14/1 -> "Wind 60KW, 50HZ, 440V7"/1("Gen Speed ")
  Constant15/1 -> "Wind 60KW, 50HZ, 440V7"/2(PA (deg))
  Constant16/1 -> "Wind 60KW, 50HZ, 440V7"/3(Wind Speed (m/s))
  Constant17/1 -> "Wind 60KW, 50HZ, 440V8"/1("Gen Speed ")
  Constant18/1 -> "Wind 60KW, 50HZ, 440V8"/2(PA (deg))
  Constant19/1 -> "Wind 60KW, 50HZ, 440V8"/3(Wind Speed (m/s))
  Constant33/1 -> "Wind 60KW, 50HZ, 440V9"/1("Gen Speed ")
  Constant34/1 -> "Wind 60KW, 50HZ, 440V9"/2(PA (deg))
  Constant35/1 -> "Wind 60KW, 50HZ, 440V9"/3(Wind Speed (m/s))
  Constant25/1 -> "Wind 60KW, 50HZ, 440V10"/1("Gen Speed ")
  Constant32/1 -> "Wind 60KW, 50HZ, 440V10"/2(PA (deg))
  Constant36/1 -> "Wind 60KW, 50HZ, 440V10"/3(Wind Speed (m/s))
  Constant26/1 -> "Wind 60KW, 50HZ, 440V11"/1("Gen Speed ")
  Constant27/1 -> "Wind 60KW, 50HZ, 440V11"/2(PA (deg))
  Constant28/1 -> "Wind 60KW, 50HZ, 440V11"/3(Wind Speed (m/s))
  Constant29/1 -> "Wind 60KW, 50HZ, 440V12"/1("Gen Speed ")
  Constant30/1 -> "Wind 60KW, 50HZ, 440V12"/2(PA (deg))
  Constant31/1 -> "Wind 60KW, 50HZ, 440V12"/3(Wind Speed (m/s))
  Constant45/1 -> "Wind 60KW, 50HZ, 440V16"/1("Gen Speed ")
  Constant46/1 -> "Wind 60KW, 50HZ, 440V16"/2(PA (deg))
  Constant47/1 -> "Wind 60KW, 50HZ, 440V16"/3(Wind Speed (m/s))
  Constant37/1 -> "Wind 60KW, 50HZ, 440V13"/1("Gen Speed ")
  Constant44/1 -> "Wind 60KW, 50HZ, 440V13"/2(PA (deg))
  Constant48/1 -> "Wind 60KW, 50HZ, 440V13"/3(Wind Speed (m/s))
  Constant38/1 -> "Wind 60KW, 50HZ, 440V14"/1("Gen Speed ")
  Constant39/1 -> "Wind 60KW, 50HZ, 440V14"/2(PA (deg))
  Constant40/1 -> "Wind 60KW, 50HZ, 440V14"/3(Wind Speed (m/s))
  Constant41/1 -> "Wind 60KW, 50HZ, 440V15"/1("Gen Speed ")
  Constant42/1 -> "Wind 60KW, 50HZ, 440V15"/2(PA (deg))
  Constant43/1 -> "Wind 60KW, 50HZ, 440V15"/3(Wind Speed (m/s))
  Constant57/1 -> "Wind 60KW, 50HZ, 440V20"/1("Gen Speed ")
  Constant58/1 -> "Wind 60KW, 50HZ, 440V20"/2(PA (deg))
  Constant59/1 -> "Wind 60KW, 50HZ, 440V20"/3(Wind Speed (m/s))
  Constant49/1 -> "Wind 60KW, 50HZ, 440V17"/1("Gen Speed ")
  Constant56/1 -> "Wind 60KW, 50HZ, 440V17"/2(PA (deg))
  Constant60/1 -> "Wind 60KW, 50HZ, 440V17"/3(Wind Speed (m/s))
  Constant50/1 -> "Wind 60KW, 50HZ, 440V18"/1("Gen Speed ")
  Constant51/1 -> "Wind 60KW, 50HZ, 440V18"/2(PA (deg))
  Constant52/1 -> "Wind 60KW, 50HZ, 440V18"/3(Wind Speed (m/s))
  Constant53/1 -> "Wind 60KW, 50HZ, 440V19"/1("Gen Speed ")
  Constant54/1 -> "Wind 60KW, 50HZ, 440V19"/2(PA (deg))
  Constant55/1 -> "Wind 60KW, 50HZ, 440V19"/3(Wind Speed (m/s))
  connections:
  "Wind 60KW, 50HZ, 440V22"/RConn1 -- "Wind 60KW, 50HZ, 440V2"/RConn1 -- "Wind 60KW, 50HZ, 440V1"/RConn1 -- "Wind 60KW, 50HZ, 440V3"/RConn1 -- "Wind 60KW, 50HZ, 440V4"/RConn1 -- "Wind 60KW, 50HZ, 440V8"/RConn1 -- "Wind 60KW, 50HZ, 440V7"/RConn1 -- "Wind 60KW, 50HZ, 440V5"/RConn1 -- "Wind 60KW, 50HZ, 440V6"/RConn1 -- "Wind 60KW, 50HZ, 440V9"/RConn1 -- "Wind 60KW, 50HZ, 440V10"/RConn1 -- "Wind 60KW, 50HZ, 440V11"/RConn1 -- "Wind 60KW, 50HZ, 440V12"/RConn1 -- "Wind 60KW, 50HZ, 440V15"/RConn1 -- "Wind 60KW, 50HZ, 440V14"/RConn1 -- "Wind 60KW, 50HZ, 440V13"/RConn1 -- "Wind 60KW, 50HZ, 440V16"/RConn1 -- a/RConn1 -- "Wind 60KW, 50HZ, 440V19"/RConn1 -- "Wind 60KW, 50HZ, 440V18"/RConn1 -- "Wind 60KW, 50HZ, 440V17"/RConn1 -- "Wind 60KW, 50HZ, 440V20"/RConn1 -- "Wind 60KW, 50HZ, 440V24"/RConn1 -- "Wind 60KW, 50HZ, 440V23"/RConn1 -- "Wind 60KW, 50HZ, 440V21"/RConn1 -- "Wind 60KW, 50HZ, 440V25"/RConn1
  "Wind 60KW, 50HZ, 440V22"/RConn2 -- "Wind 60KW, 50HZ, 440V1"/RConn2 -- "Wind 60KW, 50HZ, 440V2"/RConn2 -- "Wind 60KW, 50HZ, 440V3"/RConn2 -- "Wind 60KW, 50HZ, 440V4"/RConn2 -- "Wind 60KW, 50HZ, 440V8"/RConn2 -- "Wind 60KW, 50HZ, 440V7"/RConn2 -- "Wind 60KW, 50HZ, 440V5"/RConn2 -- "Wind 60KW, 50HZ, 440V6"/RConn2 -- "Wind 60KW, 50HZ, 440V9"/RConn2 -- "Wind 60KW, 50HZ, 440V10"/RConn2 -- "Wind 60KW, 50HZ, 440V11"/RConn2 -- "Wind 60KW, 50HZ, 440V12"/RConn2 -- "Wind 60KW, 50HZ, 440V15"/RConn2 -- "Wind 60KW, 50HZ, 440V14"/RConn2 -- "Wind 60KW, 50HZ, 440V16"/RConn2 -- "Wind 60KW, 50HZ, 440V13"/RConn2 -- b/RConn1 -- "Wind 60KW, 50HZ, 440V19"/RConn2 -- "Wind 60KW, 50HZ, 440V18"/RConn2 -- "Wind 60KW, 50HZ, 440V20"/RConn2 -- "Wind 60KW, 50HZ, 440V17"/RConn2 -- "Wind 60KW, 50HZ, 440V24"/RConn2 -- "Wind 60KW, 50HZ, 440V23"/RConn2 -- "Wind 60KW, 50HZ, 440V21"/RConn2 -- "Wind 60KW, 50HZ, 440V25"/RConn2
  "Wind 60KW, 50HZ, 440V22"/RConn3 -- "Wind 60KW, 50HZ, 440V23"/RConn3 -- "Wind 60KW, 50HZ, 440V1"/RConn3 -- "Wind 60KW, 50HZ, 440V2"/RConn3 -- "Wind 60KW, 50HZ, 440V3"/RConn3 -- "Wind 60KW, 50HZ, 440V4"/RConn3 -- "Wind 60KW, 50HZ, 440V8"/RConn3 -- "Wind 60KW, 50HZ, 440V7"/RConn3 -- "Wind 60KW, 50HZ, 440V5"/RConn3 -- "Wind 60KW, 50HZ, 440V6"/RConn3 -- "Wind 60KW, 50HZ, 440V9"/RConn3 -- "Wind 60KW, 50HZ, 440V10"/RConn3 -- "Wind 60KW, 50HZ, 440V11"/RConn3 -- "Wind 60KW, 50HZ, 440V12"/RConn3 -- "Wind 60KW, 50HZ, 440V15"/RConn3 -- "Wind 60KW, 50HZ, 440V14"/RConn3 -- "Wind 60KW, 50HZ, 440V16"/RConn3 -- "Wind 60KW, 50HZ, 440V13"/RConn3 -- c/RConn1 -- "Wind 60KW, 50HZ, 440V19"/RConn3 -- "Wind 60KW, 50HZ, 440V18"/RConn3 -- "Wind 60KW, 50HZ, 440V20"/RConn3 -- "Wind 60KW, 50HZ, 440V17"/RConn3 -- "Wind 60KW, 50HZ, 440V24"/RConn3 -- "Wind 60KW, 50HZ, 440V25"/RConn3 -- "Wind 60KW, 50HZ, 440V21"/RConn3

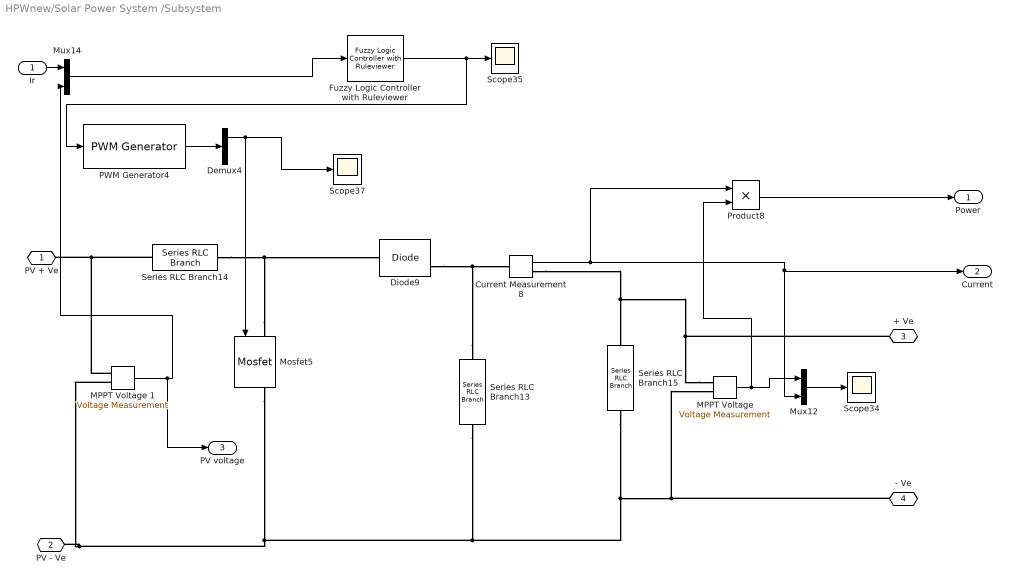
== system HPWnew/Solar Power System /Subsystem ==
  Ir : Inport
  Current Measurement8 : powerlib/Measurements/Current Measurement  PhasorSimulation=off  OutputType=Complex  PSBequivalent=0
  Demux4 : Demux  Outputs=2
  Diode9 : powerlib/Power Electronics/Diode  Ron=0.001  Lon=0  Vf=0.8  IC=0  UseSnubber=off  Rs=500  Cs=250e-9  Measurements=on
  Fuzzy Logic Controller with Ruleviewer : fuzblock/Fuzzy Logic  Controller  with Ruleviewer  fismatrix=[PV1]  Ts=0.1
  "MPPT Voltage " : powerlib/Measurements/Voltage Measurement  PhasorSimulation=off  OutputType=Complex  PSBequivalent=0
  MPPT Voltage 1 : powerlib/Measurements/Voltage Measurement  PhasorSimulation=off  OutputType=Complex  PSBequivalent=0
  Mosfet5 : powerlib/Power Electronics/Mosfet  Ron=0.1  Lon=0  Rd=0.01  Vfd=0  IC=0  Rs=1e5  Cs=inf  Measurements=on
  Mux12 : Mux  Inputs=2
  Mux14 : Mux  Inputs=2
  PWM Generator4 : powerlib_extras/Control  Blocks/PWM Generator  GeneratorMode="1-arm  bridge (2 pulses)"  Fc=2000  Internal=off  mIndex=0.4  Freq=50  Phase=0
  Product8 : Product  RndMeth=Zero
  Scope34 : Scope
      settings: ShowLegends=on  YMin=0  YMax=70  MaxDataPoints=50000000
  Scope35 : Scope
      settings: YMin=0.608449  YMax=0.672497  SaveName=ScopeData2  MaxDataPoints=50000000
  Scope37 : Scope
      settings: YMin=18.82  YMax=18.95  SaveName=ScopeData4  MaxDataPoints=50000000
  Series RLC Branch13 : powerlib/Elements/Series RLC Branch  LConnTagsString=__new0  RConnTagsString=__new0  BranchType=C  Resistance=1  Inductance=1e-3  SetiL0=off  InitialCurrent=0  Capacitance=550e-6  Setx0=off  InitialVoltage=0  Measurements=None
  Series RLC Branch14 : powerlib/Elements/Series RLC Branch  LConnTagsString=__new0  RConnTagsString=__new0  BranchType=L  Resistance=1  Inductance=161e-3  SetiL0=off  InitialCurrent=0  Capacitance=1e-6  Setx0=off  InitialVoltage=0  Measurements=None
  Series RLC Branch15 : powerlib/Elements/Series RLC Branch  LConnTagsString=__new0  RConnTagsString=__new0  BranchType=R  Resistance=110  Inductance=1e-3  SetiL0=off  InitialCurrent=0  Capacitance=1e-6  Setx0=off  InitialVoltage=0  Measurements=None
  PV + Ve : PMIOPort  Port=1  Side=Left
  PV - Ve : PMIOPort  Port=2  Side=Left
  + Ve : PMIOPort  Port=3  Side=Right
  - Ve : PMIOPort  Port=4  Side=Right
  Power : Outport
  "Current " : Outport  Port=2
  "PV voltage " : Outport  Port=3
  wires:
  Current Measurement8/1 -> "Current "/1, Mux12/2, Product8/1
  "MPPT Voltage "/1 -> Mux12/1, Product8/2
  Mux12/1 -> Scope34/1
  Product8/1 -> Power/1
  Fuzzy Logic Controller with Ruleviewer/1 -> PWM Generator4/1, Scope35/1
  Mux14/1 -> Fuzzy Logic Controller with Ruleviewer/1
  Demux4/1 -> Mosfet5/1, Scope37/1
  PWM Generator4/1 -> Demux4/1
  Ir/1 -> Mux14/1
  MPPT Voltage 1/1 -> "PV voltage "/1, Mux14/2
  connections:
  Mosfet5/LConn1 -- Diode9/LConn1 -- Series RLC Branch14/RConn1
  Series RLC Branch13/LConn1 -- Current Measurement8/LConn1 -- Diode9/RConn1
  "MPPT Voltage "/LConn1 -- Current Measurement8/RConn1 -- Series RLC Branch15/LConn1 -- + Ve/RConn1
  Mosfet5/RConn1 -- Series RLC Branch15/RConn1 -- "MPPT Voltage "/LConn2 -- - Ve/RConn1 -- Series RLC Branch13/RConn1 -- PV - Ve/RConn1 -- MPPT Voltage 1/LConn2
  PV + Ve/RConn1 -- Series RLC Branch14/LConn1 -- MPPT Voltage 1/LConn1

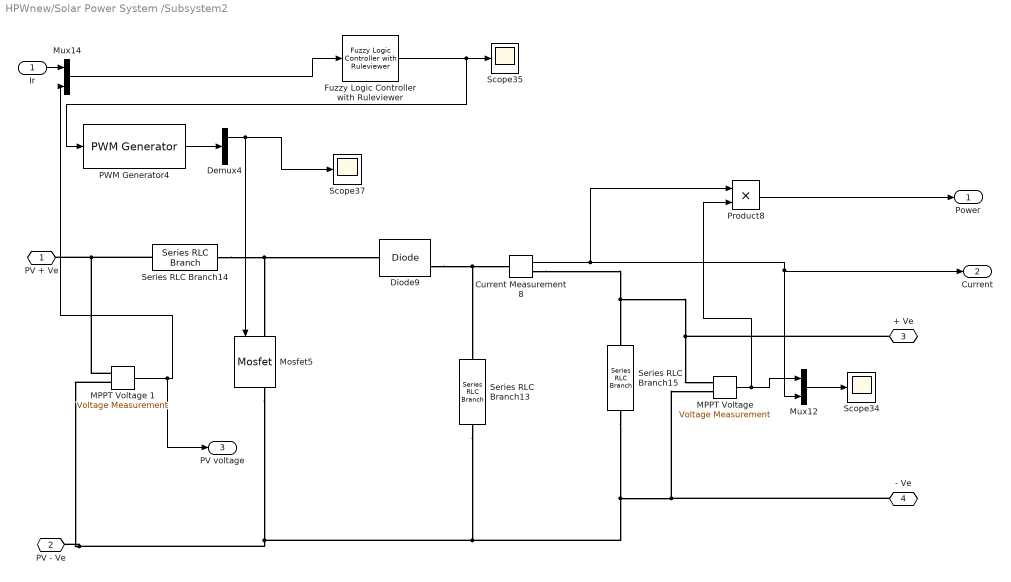
== system HPWnew/Solar Power System /Subsystem2 ==
  Ir : Inport
  Current Measurement8 : powerlib/Measurements/Current Measurement  PhasorSimulation=off  OutputType=Complex  PSBequivalent=0
  Demux4 : Demux  Outputs=2
  Diode9 : powerlib/Power Electronics/Diode  Ron=0.001  Lon=0  Vf=0.8  IC=0  UseSnubber=off  Rs=500  Cs=250e-9  Measurements=on
  Fuzzy Logic Controller with Ruleviewer : fuzblock/Fuzzy Logic  Controller  with Ruleviewer  fismatrix=[PV2]  Ts=0.1
  "MPPT Voltage " : powerlib/Measurements/Voltage Measurement  PhasorSimulation=off  OutputType=Complex  PSBequivalent=0
  MPPT Voltage 1 : powerlib/Measurements/Voltage Measurement  PhasorSimulation=off  OutputType=Complex  PSBequivalent=0
  Mosfet5 : powerlib/Power Electronics/Mosfet  Ron=0.1  Lon=0  Rd=0.01  Vfd=0  IC=0  Rs=1e5  Cs=inf  Measurements=on
  Mux12 : Mux  Inputs=2
  Mux14 : Mux  Inputs=2
  PWM Generator4 : powerlib_extras/Control  Blocks/PWM Generator  GeneratorMode="1-arm  bridge (2 pulses)"  Fc=2000  Internal=off  mIndex=0.4  Freq=50  Phase=0
  Product8 : Product  RndMeth=Zero
  Scope34 : Scope
      settings: ShowLegends=on  YMin=0  YMax=70  MaxDataPoints=50000000
  Scope35 : Scope
      settings: YMin=0.608449  YMax=0.672497  SaveName=ScopeData2  MaxDataPoints=50000000
  Scope37 : Scope
      settings: YMin=18.82  YMax=18.95  SaveName=ScopeData4  MaxDataPoints=50000000
  Series RLC Branch13 : powerlib/Elements/Series RLC Branch  LConnTagsString=__new0  RConnTagsString=__new0  BranchType=C  Resistance=1  Inductance=1e-3  SetiL0=off  InitialCurrent=0  Capacitance=550e-6  Setx0=off  InitialVoltage=0  Measurements=None
  Series RLC Branch14 : powerlib/Elements/Series RLC Branch  LConnTagsString=__new0  RConnTagsString=__new0  BranchType=L  Resistance=1  Inductance=161e-3  SetiL0=off  InitialCurrent=0  Capacitance=1e-6  Setx0=off  InitialVoltage=0  Measurements=None
  Series RLC Branch15 : powerlib/Elements/Series RLC Branch  LConnTagsString=__new0  RConnTagsString=__new0  BranchType=R  Resistance=110  Inductance=1e-3  SetiL0=off  InitialCurrent=0  Capacitance=1e-6  Setx0=off  InitialVoltage=0  Measurements=None
  PV + Ve : PMIOPort  Port=1  Side=Left
  PV - Ve : PMIOPort  Port=2  Side=Left
  + Ve : PMIOPort  Port=3  Side=Right
  - Ve : PMIOPort  Port=4  Side=Right
  Power : Outport
  "Current " : Outport  Port=2
  "PV voltage " : Outport  Port=3
  wires:
  MPPT Voltage 1/1 -> Mux14/2, "PV voltage "/1
  Ir/1 -> Mux14/1
  PWM Generator4/1 -> Demux4/1
  Demux4/1 -> Scope37/1, Mosfet5/1
  Mux14/1 -> Fuzzy Logic Controller with Ruleviewer/1
  Fuzzy Logic Controller with Ruleviewer/1 -> Scope35/1, PWM Generator4/1
  Product8/1 -> Power/1
  Mux12/1 -> Scope34/1
  "MPPT Voltage "/1 -> Product8/2, Mux12/1
  Current Measurement8/1 -> Product8/1, Mux12/2, "Current "/1
  connections:
  MPPT Voltage 1/LConn1 -- Series RLC Branch14/LConn1 -- PV + Ve/RConn1
  MPPT Voltage 1/LConn2 -- PV - Ve/RConn1 -- Series RLC Branch13/RConn1 -- - Ve/RConn1 -- "MPPT Voltage "/LConn2 -- Series RLC Branch15/RConn1 -- Mosfet5/RConn1
  + Ve/RConn1 -- Series RLC Branch15/LConn1 -- Current Measurement8/RConn1 -- "MPPT Voltage "/LConn1
  Diode9/RConn1 -- Current Measurement8/LConn1 -- Series RLC Branch13/LConn1
  Series RLC Branch14/RConn1 -- Diode9/LConn1 -- Mosfet5/LConn1

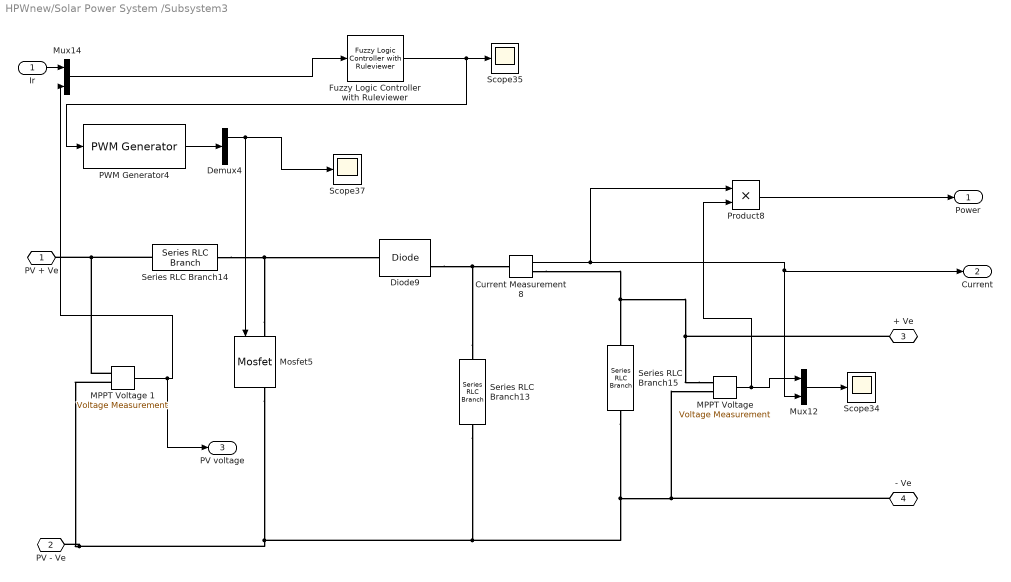
== system HPWnew/Solar Power System /Subsystem3 ==
  Ir : Inport
  Current Measurement8 : powerlib/Measurements/Current Measurement  PhasorSimulation=off  OutputType=Complex  PSBequivalent=0
  Demux4 : Demux  Outputs=2
  Diode9 : powerlib/Power Electronics/Diode  Ron=0.001  Lon=0  Vf=0.8  IC=0  UseSnubber=off  Rs=500  Cs=250e-9  Measurements=on
  Fuzzy Logic Controller with Ruleviewer : fuzblock/Fuzzy Logic  Controller  with Ruleviewer  fismatrix=[PV3]  Ts=0.1
  "MPPT Voltage " : powerlib/Measurements/Voltage Measurement  PhasorSimulation=off  OutputType=Complex  PSBequivalent=0
  MPPT Voltage 1 : powerlib/Measurements/Voltage Measurement  PhasorSimulation=off  OutputType=Complex  PSBequivalent=0
  Mosfet5 : powerlib/Power Electronics/Mosfet  Ron=0.1  Lon=0  Rd=0.01  Vfd=0  IC=0  Rs=1e5  Cs=inf  Measurements=on
  Mux12 : Mux  Inputs=2
  Mux14 : Mux  Inputs=2
  PWM Generator4 : powerlib_extras/Control  Blocks/PWM Generator  GeneratorMode="1-arm  bridge (2 pulses)"  Fc=2000  Internal=off  mIndex=0.4  Freq=50  Phase=0
  Product8 : Product  RndMeth=Zero
  Scope34 : Scope
      settings: ShowLegends=on  YMin=0  YMax=70  MaxDataPoints=50000000
  Scope35 : Scope
      settings: YMin=0.608449  YMax=0.672497  SaveName=ScopeData2  MaxDataPoints=50000000
  Scope37 : Scope
      settings: YMin=18.82  YMax=18.95  SaveName=ScopeData4  MaxDataPoints=50000000
  Series RLC Branch13 : powerlib/Elements/Series RLC Branch  LConnTagsString=__new0  RConnTagsString=__new0  BranchType=C  Resistance=1  Inductance=1e-3  SetiL0=off  InitialCurrent=0  Capacitance=550e-6  Setx0=off  InitialVoltage=0  Measurements=None
  Series RLC Branch14 : powerlib/Elements/Series RLC Branch  LConnTagsString=__new0  RConnTagsString=__new0  BranchType=L  Resistance=1  Inductance=161e-3  SetiL0=off  InitialCurrent=0  Capacitance=1e-6  Setx0=off  InitialVoltage=0  Measurements=None
  Series RLC Branch15 : powerlib/Elements/Series RLC Branch  LConnTagsString=__new0  RConnTagsString=__new0  BranchType=R  Resistance=110  Inductance=1e-3  SetiL0=off  InitialCurrent=0  Capacitance=1e-6  Setx0=off  InitialVoltage=0  Measurements=None
  PV + Ve : PMIOPort  Port=1  Side=Left
  PV - Ve : PMIOPort  Port=2  Side=Left
  + Ve : PMIOPort  Port=3  Side=Right
  - Ve : PMIOPort  Port=4  Side=Right
  Power : Outport
  "Current " : Outport  Port=2
  "PV voltage " : Outport  Port=3
  wires:
  Current Measurement8/1 -> "Current "/1, Mux12/2, Product8/1
  "MPPT Voltage "/1 -> Mux12/1, Product8/2
  Mux12/1 -> Scope34/1
  Product8/1 -> Power/1
  Fuzzy Logic Controller with Ruleviewer/1 -> PWM Generator4/1, Scope35/1
  Mux14/1 -> Fuzzy Logic Controller with Ruleviewer/1
  Demux4/1 -> Mosfet5/1, Scope37/1
  PWM Generator4/1 -> Demux4/1
  Ir/1 -> Mux14/1
  MPPT Voltage 1/1 -> "PV voltage "/1, Mux14/2
  connections:
  Mosfet5/LConn1 -- Diode9/LConn1 -- Series RLC Branch14/RConn1
  Series RLC Branch13/LConn1 -- Current Measurement8/LConn1 -- Diode9/RConn1
  "MPPT Voltage "/LConn1 -- Current Measurement8/RConn1 -- Series RLC Branch15/LConn1 -- + Ve/RConn1
  Mosfet5/RConn1 -- Series RLC Branch15/RConn1 -- "MPPT Voltage "/LConn2 -- - Ve/RConn1 -- Series RLC Branch13/RConn1 -- PV - Ve/RConn1 -- MPPT Voltage 1/LConn2
  PV + Ve/RConn1 -- Series RLC Branch14/LConn1 -- MPPT Voltage 1/LConn1

== system HPWnew/Solar Power System /VSC1 Control ==
  note: VSC Main Controller
  Vabc_prim : Inport  PortDimensions=3
  Iabc_prim : Inport  Port=2  PortDimensions=3
  Vdc_mes : Inport  Port=3  PortDimensions=1
  Current Regulator : Subsystem
  Gain : Gain  Gain=-1
  Iq_ref : Constant  Value=0
  Mux : Mux  Inputs=2
  PLL & Measurements : Subsystem
  Uabc_ref Generation max (m) = 1 : Subsystem
  VDC Regulator : Subsystem
  Vdc_ref1 : Constant  Value=Vdc_ref
  Uref : Outport
  wires:
  Vdc_ref1/1 -> VDC Regulator/2(Vdc_ref)
  Uabc_ref Generation max (m) = 1/1(Uabc_ref) -> Uref/1
  Iabc_prim/1 -> Gain/1
  Vabc_prim/1 -> PLL & Measurements/1(Vabc_prim)
  Vdc_mes/1 -> VDC Regulator/1(Vdc_mes)
  PLL & Measurements/2(VdVq_prim) -> Current Regulator/1(VdVq_mes)
  PLL & Measurements/3(IdIq_prim) -> Current Regulator/2(IdIq_mes)
  Mux/1 -> Current Regulator/3(IdIq_ref)
  Iq_ref/1 -> Mux/2
  Current Regulator/1(VdVq_conv) -> Uabc_ref Generation max (m) = 1/2(VdVq_conv)
  PLL & Measurements/1(wt) -> Uabc_ref Generation max (m) = 1/1(wt)
  VDC Regulator/1(Id_ref) -> Mux/1
  Gain/1 -> PLL & Measurements/2(Iabc_prim)
